simulink model "pidsg"  (R2020a)
settings: Solver=VariableStepAuto  StartTime=0.0  StopTime=0.15  RelTol=1e-3
values from neighbouring files (symbols this model uses):
  aiw_G = 1    [pid_sysgen_v1_0_setup.m]
  f_filter = 5000    [pid_sysgen_v1_0_setup.m]
  FPGA_CLK_MHZ = 125    [pid_sysgen_v1_0_setup.m]
  G1D = (2*R-1)/(2*R+1)    (= 0.995012468828)    [pid_sysgen_v1_0_setup.m]
  G2D = Gd/(2*R+1)    (= 498.753117207)    [pid_sysgen_v1_0_setup.m]
  Gi = ki*Ts/2    (= 1e-06)    [pid_sysgen_v1_0_setup.m]
  input_threshold = 0.0    (= 0)    [pid_sysgen_v1_0_setup.m]
  kd = 0.1    [pid_sysgen_v1_0_setup.m]
  ki = 2    [pid_sysgen_v1_0_setup.m]
  kp = 7    [pid_sysgen_v1_0_setup.m]
  max_control = 0.9    [pid_sysgen_v1_0_setup.m]
  SampleRate = 1e6    (= 1000000)    [pid_sysgen_v1_0_setup.m]
  Ts = 1/SampleRate    (= 1e-06)    [pid_sysgen_v1_0_setup.m]
  VHDL_latency_cycles = 1    [pid_sysgen_v1_0_setup.m]
libraries: xbsIndex_r4 x70, simulink x2
settings Model: Creator=osboxes  LastModifiedBy=valbas

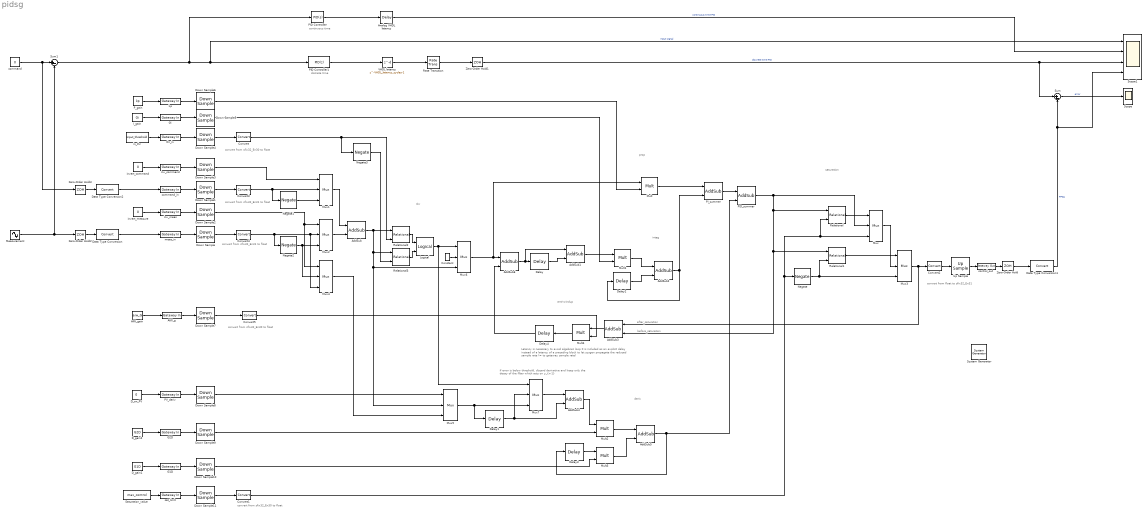
== system pidsg ==
  note: saturation
  note: convert from sfix32_En30 to float
  note: anti-windup
  note: continuous time
  note: before_saturation
  note: integ
  note: thr
  note: prop
  note: if error is below threshold, discard derivative and keep only
      | the decay of the filter which acts on y_{n-1}
  note: Latency is necessary to avoid algebraic loop
      | It is included as an explicit delay instead of a latency of a preceding block
      | to let sysgen propagate the reduced sample rate (= to gateway sample rate)
  note: convert from float to sfix32_En31
  note: convert from sfix32_En30 to float
  note: after_saturation
  note: convert from sfix32_En31 to float
  note: discrete time
  note: convert from sfix32_En31 to float
  note: deriv
  note: convert from sfix32_En30 to float
  " System Generator" : xbsIndex_r4/ System Generator  Tag=genX  xilinxfamily=zynq  part=xc7z030  speed=-1  package=sbg485  synthesis_tool=Vivado  clock_wrapper=Clock Enables  directory=./netlist  proj_type=Vivado  Synth_file=Vivado Synthesis Defaults  Impl_file=Vivado Implementation Defaults  testbench=off  simulink_period=1/(FPGA_CLK_MHZ*1.e6)  sysclk_period=1.e3/FPGA_CLK_MHZ  dcm_input_clock_period=10  incr_netlist=off  trim_vbits=Everywhere in SubSystem  dbl_ovrd=According to Block Masks  core_generation=According to Block Masks  run_coregen=off  deprecated_control=off  eval_field=0  block_type=sysgen
  AIW_g : xbsIndex_r4/Gateway In  gui_display_data_type=Fixed-point  arith_type="Signed  (2's comp)"  n_bits=32  bin_pt=30  preci_type=Single  exp_width=8  frac_width=24  rows=1  columns=1  quantization="Round  (unbiased: +/- Inf)"  overflow=Saturate  period=1/(FPGA_CLK_MHZ*1.e6)  UseAsADC=off  ADCChannel='1'  interface=None  automatic_assignment=on  address_offset=hex2dec('00')  intf_name=''  intf_description=''  default_value=0  timing_constraint=None  locs_specified=off  LOCs={}  io_standard={}  inherit_from_input=off  hdl_port=on  dbl_ovrd=off  block_type=gatewayin
  AIW_gain : Constant  Value=aiw_G  OutDataTypeStr=fixdt(1,32,30)  SampleTime=1/(FPGA_CLK_MHZ*1.e6)
  AddSub : xbsIndex_r4/AddSub  mode=Subtraction  use_carryin=off  use_carryout=off  en=off  latency=0  precision=Full  arith_type=Unsigned  n_bits=16  bin_pt=14  quantization=Truncate  overflow=Wrap  use_behavioral_HDL=off  hw_selection=Fabric  pipelined=off  dbl_ovrd=off  block_type=addsub
  AddSub{1..2,5..6} (4 alike) : xbsIndex_r4/AddSub  mode=Addition  use_carryin=off  use_carryout=off  en=off  latency=0  precision=Full  arith_type=Unsigned  n_bits=16  bin_pt=14  quantization=Truncate  overflow=Wrap  use_behavioral_HDL=off  hw_selection=Fabric  pipelined=off  dbl_ovrd=off  block_type=addsub
  AddSub3 : xbsIndex_r4/AddSub  mode=Subtraction  use_carryin=off  use_carryout=off  en=off  latency=0  precision=Full  arith_type=Unsigned  n_bits=16  bin_pt=14  quantization=Truncate  overflow=Wrap  use_behavioral_HDL=off  hw_selection=Fabric  pipelined=off  dbl_ovrd=off  block_type=addsub
  AddSub4 : xbsIndex_r4/AddSub  mode=Subtraction  use_carryin=off  use_carryout=off  en=off  latency=0  precision=Full  arith_type=Unsigned  n_bits=16  bin_pt=14  quantization=Truncate  overflow=Wrap  use_behavioral_HDL=off  hw_selection=Fabric  pipelined=off  dbl_ovrd=off  block_type=addsub
  Analog VHDL latency : TransportDelay  DelayTime=VHDL_latency_cycles*Ts
  Constant : xbsIndex_r4/Constant  const=0  gui_display_data_type=Floating-point  arith_type=Floating-point  n_bits=16  bin_pt=14  preci_type=Single  exp_width=8  frac_width=24  explicit_period=off  period=1  equ=P=C  opselect=C  inp2=PCIN>>17  opr=+  inp1=P  carry=CIN  dbl_ovrd=off  block_type=constant
  Convert{,1,3..5} (5 alike) : xbsIndex_r4/Convert  gui_display_data_type=Floating-point  arith_type=Floating-point  n_bits=16  bin_pt=14  float_type=Single  exp_bits=8  fraction_bits=24  quantization=Truncate  overflow=Wrap  en=off  latency=0  pipeline=off  dbl_ovrd=off  block_type=convert
  Convert2 : xbsIndex_r4/Convert  gui_display_data_type=Fixed-point  arith_type="Signed  (2's comp)"  n_bits=32  bin_pt=31  float_type=Single  exp_bits=8  fraction_bits=24  quantization="Round  (unbiased: +/- Inf)"  overflow=Saturate  en=off  latency=0  pipeline=off  dbl_ovrd=off  block_type=convert
  D_gain1 : Constant  Value=G1D  OutDataTypeStr=double  SampleTime=1/(FPGA_CLK_MHZ*1.e6)
  D_gain2 : Constant  Value=G2D  OutDataTypeStr=double  SampleTime=1/(FPGA_CLK_MHZ*1.e6)
  D_on_PV : Constant  Value=0  OutDataTypeStr=boolean  SampleTime=1/(FPGA_CLK_MHZ*1.e6)
  Data Type Conversion : DataTypeConversion
  Data Type Conversion1 : DataTypeConversion
  Data Type Conversion2 : DataTypeConversion
  Delay{,1..4} (5 alike) : xbsIndex_r4/Delay  rst=off  infoeditControl=Selection of Reset will increase slice count due to use of real FFs and instead of SRLs  en=off  latency=1  reg_retiming=off  dbl_ovrd=off  block_type=delay
  Down Sample{,1..11} (12 alike) : xbsIndex_r4/Down Sample  sample_ratio=FPGA_CLK_MHZ*1.e6/SampleRate  sample_phase="Last Value of Frame  (most efficient)"  en=off  rst=off  latency=1  dbl_ovrd=off  block_type=dsamp
  G1D : xbsIndex_r4/Gateway In  gui_display_data_type=Floating-point  arith_type=Floating-point  n_bits=16  bin_pt=14  preci_type=Single  exp_width=8  frac_width=24  rows=1  columns=1  quantization="Round  (unbiased: +/- Inf)"  overflow=Saturate  period=1/(FPGA_CLK_MHZ*1.e6)  UseAsADC=off  ADCChannel='1'  interface=None  automatic_assignment=on  address_offset=hex2dec('00')  intf_name=''  intf_description=''  default_value=0  timing_constraint=None  locs_specified=off  LOCs={}  io_standard={}  inherit_from_input=off  hdl_port=on  dbl_ovrd=off  block_type=gatewayin
  G2D : xbsIndex_r4/Gateway In  gui_display_data_type=Floating-point  arith_type=Floating-point  n_bits=16  bin_pt=14  preci_type=Single  exp_width=8  frac_width=24  rows=1  columns=1  quantization="Round  (unbiased: +/- Inf)"  overflow=Saturate  period=1/(FPGA_CLK_MHZ*1.e6)  UseAsADC=off  ADCChannel='1'  interface=None  automatic_assignment=on  address_offset=hex2dec('00')  intf_name=''  intf_description=''  default_value=0  timing_constraint=None  locs_specified=off  LOCs={}  io_standard={}  inherit_from_input=off  hdl_port=on  dbl_ovrd=off  block_type=gatewayin
  Gi : xbsIndex_r4/Gateway In  gui_display_data_type=Floating-point  arith_type=Floating-point  n_bits=16  bin_pt=14  preci_type=Single  exp_width=8  frac_width=24  rows=1  columns=1  quantization="Round  (unbiased: +/- Inf)"  overflow=Saturate  period=1/(FPGA_CLK_MHZ*1.e6)  UseAsADC=off  ADCChannel='1'  interface=None  automatic_assignment=on  address_offset=hex2dec('00')  intf_name=''  intf_description=''  default_value=0  timing_constraint=None  locs_specified=off  LOCs={}  io_standard={}  inherit_from_input=off  hdl_port=on  dbl_ovrd=off  block_type=gatewayin
  I_gain : Constant  Value=Gi  OutDataTypeStr=double  SampleTime=1/(FPGA_CLK_MHZ*1.e6)
  Logical : xbsIndex_r4/Logical  logical_function=OR  inputs=2  en=off  latency=0  precision=Full  arith_type=Unsigned  n_bits=16  bin_pt=0  align_bp=on  dbl_ovrd=off  block_type=logical
  Measurement : Sin  Amplitude=0.1  Frequency=2*pi*17  Phase=0*pi  SampleTime=0
  Mult{,1..4} (5 alike) : xbsIndex_r4/Mult  precision=Full  arith_type="Signed  (2's comp)"  n_bits=16  bin_pt=14  quantization=Truncate  overflow=Wrap  en=off  latency=0  use_behavioral_HDL=off  opt=Speed  use_embedded=on  optimum_pipeline=off  pipeline=on  dbl_ovrd=off  use_rpm=on  placement_style=Triangular  block_type=mult
  Mux{,1..7} (8 alike) : xbsIndex_r4/Mux  inputs=2  en=off  latency=0  precision=Full  arith_type=Unsigned  n_bits=16  bin_pt=14  quantization=Truncate  overflow=Wrap  dbl_ovrd=off  block_type=mux
  Negate{,1..3} (4 alike) : xbsIndex_r4/Negate  precision=Full  arith_type=Unsigned  n_bits=16  bin_pt=14  quantization=Truncate  overflow=Wrap  en=off  latency=0  dbl_ovrd=off  block_type=negate
  PID Controller : simulink/Continuous/PID Controller  Controller=PID  Form=Parallel  TimeDomain=Continuous-time  UseExternalTs=off  SampleTime=-1  IntegratorMethod=Forward Euler  FilterMethod=Forward Euler  ControllerParametersSource=internal  P=kp  I=ki  D=kd  UseFilter=on  N=f_filter  TunerSelectOption=Transfer Function Based (PID Tuner App)  InitialConditionSource=internal  InitialConditionForIntegrator=0  InitialConditionForFilter=0  DifferentiatorICPrevScaledInput=0  ExternalReset=none  TrackingMode=off  Kt=1  LimitOutput=off  UpperSaturationLimit=inf  LowerSaturationLimit=-inf  LinearizeAsGain=on  AntiWindupMode=none  Kb=1  POutMin=[]  POutMax=[]  IOutMin=[]  IOutMax=[]  DOutMin=[]  DOutMax=[]  NOutMin=[]  NOutMax=[]  SumOutMin=[]  SumOutMax=[]  SaturationOutMin=[]  SaturationOutMax=[]  PParamMin=[]  PParamMax=[]  IParamMin=[]  IParamMax=[]  DParamMin=[]  DParamMax=[]  NParamMin=[]  NParamMax=[]  KbParamMin=[]  KbParamMax=[]  KtParamMin=[]  KtParamMax=[]  KbOutMin=[]  KbOutMax=[]  KtOutMin=[]  KtOutMax=[]  IntegratorOutMin=[]  IntegratorOutMax=[]  FilterOutMin=[]  FilterOutMax=[]  SumI1OutMin=[]  SumI1OutMax=[]  SumI2OutMin=[]  SumI2OutMax=[]  SumI3OutMin=[]  SumI3OutMax=[]  SumI4OutMin=[]  SumI4OutMax=[]  SumDOutMin=[]  SumDOutMax=[]  DifferentiatorOutMin=[]  DifferentiatorOutMax=[]  FilterDiffOutCoefMin=[]  FilterDiffOutCoefMax=[]  ReciprocalOutMin=[]  ReciprocalOutMax=[]  SumDenOutMin=[]  SumDenOutMax=[]  SumNumOutMin=[]  SumNumOutMax=[]  DivideOutMin=[]  DivideOutMax=[]  UdiffTsProdOutMin=[]  UdiffTsProdOutMax=[]  NTsProdOutMin=[]  NTsProdOutMax=[]  UintegralTsProdOutMin=[]  UintegralTsProdOutMax=[]  UngainTsProdOutMin=[]  UngainTsProdOutMax=[]  IntegratorContinuousStateAttributes=''  IntegratorStateMustResolveToSignalObject=off  IntegratorRTWStateStorageClass=Auto  FilterContinuousStateAttributes=''  FilterStateMustResolveToSignalObject=off  FilterRTWStateStorageClass=Auto  ParallelPVariant=InternalParameters  IdealPVariant=Disabled  IVariant=InternalParameters  DVariant=InternalParameters  IntegratorVariant=Continuous  SatVariant=Disabled  AWVariant=Passthrough  PCopyVariant=Disabled  TRVariant=Disabled  FdbkBlocksVariant=Forward  IdealPFdbkVariant=Disabled  SatFdbkVariant=Disabled  DerivativeFilterVariant=ContFilter  NVariant=InternalParameters  NCopyVariant=Disabled  FilterICVariant=InternalICsFilter  IntegratorICVariant=InternalICs  ExternalResetVariant=Disabled  TRSumVariant=Passthrough  SumFdbkVariant=Disabled  SumVariant=Sum_PID  TsampFilterVariant=InternalTs  TsampNgainVariant=Passthrough  TsampIntegralVariant=Passthrough
  PID Controller1 : simulink/Continuous/PID Controller  Controller=PID  Form=Parallel  TimeDomain=Discrete-time  UseExternalTs=off  SampleTime=Ts  IntegratorMethod=Trapezoidal  FilterMethod=Trapezoidal  ControllerParametersSource=internal  P=kp  I=ki  D=kd  UseFilter=on  N=f_filter  TunerSelectOption=Transfer Function Based (PID Tuner App)  InitialConditionSource=internal  InitialConditionForIntegrator=0  InitialConditionForFilter=0  DifferentiatorICPrevScaledInput=0  ExternalReset=none  TrackingMode=off  Kt=1  LimitOutput=on  UpperSaturationLimit=max_control  LowerSaturationLimit=-max_control  LinearizeAsGain=on  AntiWindupMode=back-calculation  Kb=aiw_G*ki  POutMin=[]  POutMax=[]  IOutMin=[]  IOutMax=[]  DOutMin=[]  DOutMax=[]  NOutMin=[]  NOutMax=[]  SumOutMin=[]  SumOutMax=[]  SaturationOutMin=[]  SaturationOutMax=[]  PParamMin=[]  PParamMax=[]  IParamMin=[]  IParamMax=[]  DParamMin=[]  DParamMax=[]  NParamMin=[]  NParamMax=[]  KbParamMin=[]  KbParamMax=[]  KtParamMin=[]  KtParamMax=[]  KbOutMin=[]  KbOutMax=[]  KtOutMin=[]  KtOutMax=[]  IntegratorOutMin=[]  IntegratorOutMax=[]  FilterOutMin=[]  FilterOutMax=[]  SumI1OutMin=[]  SumI1OutMax=[]  SumI2OutMin=[]  SumI2OutMax=[]  SumI3OutMin=[]  SumI3OutMax=[]  SumI4OutMin=[]  SumI4OutMax=[]  SumDOutMin=[]  SumDOutMax=[]  DifferentiatorOutMin=[]  DifferentiatorOutMax=[]  FilterDiffOutCoefMin=[]  FilterDiffOutCoefMax=[]  ReciprocalOutMin=[]  ReciprocalOutMax=[]  SumDenOutMin=[]  SumDenOutMax=[]  SumNumOutMin=[]  SumNumOutMax=[]  DivideOutMin=[]  DivideOutMax=[]  UdiffTsProdOutMin=[]  UdiffTsProdOutMax=[]  NTsProdOutMin=[]  NTsProdOutMax=[]  UintegralTsProdOutMin=[]  UintegralTsProdOutMax=[]  UngainTsProdOutMin=[]  UngainTsProdOutMax=[]  IntegratorContinuousStateAttributes=''  IntegratorStateMustResolveToSignalObject=off  IntegratorRTWStateStorageClass=Auto  FilterContinuousStateAttributes=''  FilterStateMustResolveToSignalObject=off  FilterRTWStateStorageClass=Auto  ParallelPVariant=InternalParameters  IdealPVariant=Disabled  IVariant=InternalParameters  DVariant=InternalParameters  IntegratorVariant=Discrete  SatVariant=Enabled  AWVariant=BackCalculation  PCopyVariant=Disabled  TRVariant=Disabled  FdbkBlocksVariant=Feedback  IdealPFdbkVariant=Passthrough  SatFdbkVariant=Enabled  DerivativeFilterVariant=TrapezoidalFilter  NVariant=InternalParameters  NCopyVariant=InternalParameters  FilterICVariant=InternalICsFilter  IntegratorICVariant=InternalICs  ExternalResetVariant=Disabled  TRSumVariant=Passthrough  SumFdbkVariant=Enabled  SumVariant=Sum_PID  TsampFilterVariant=InternalTs  TsampNgainVariant=Passthrough  TsampIntegralVariant=Passthrough
  PID_summer : xbsIndex_r4/AddSub  mode=Addition  use_carryin=off  use_carryout=off  en=off  latency=0  precision=Full  arith_type=Unsigned  n_bits=16  bin_pt=14  quantization=Truncate  overflow=Wrap  use_behavioral_HDL=off  hw_selection=Fabric  pipelined=off  dbl_ovrd=off  block_type=addsub
  PI_summer : xbsIndex_r4/AddSub  mode=Addition  use_carryin=off  use_carryout=off  en=off  latency=0  precision=Full  arith_type=Unsigned  n_bits=16  bin_pt=14  quantization=Truncate  overflow=Wrap  use_behavioral_HDL=off  hw_selection=Fabric  pipelined=off  dbl_ovrd=off  block_type=addsub
  PV_deriv : xbsIndex_r4/Gateway In  gui_display_data_type=Boolean  arith_type=Boolean  n_bits=16  bin_pt=14  preci_type=Single  exp_width=8  frac_width=24  rows=1  columns=1  quantization="Round  (unbiased: +/- Inf)"  overflow=Saturate  period=1/(FPGA_CLK_MHZ*1.e6)  UseAsADC=off  ADCChannel='1'  interface=None  automatic_assignment=on  address_offset=hex2dec('00')  intf_name=''  intf_description=''  default_value=0  timing_constraint=None  locs_specified=off  LOCs={}  io_standard={}  inherit_from_input=off  hdl_port=on  dbl_ovrd=off  block_type=gatewayin
  P_gain : Constant  Value=kp  OutDataTypeStr=double  SampleTime=1/(FPGA_CLK_MHZ*1.e6)
  Rate Transition : RateTransition  OutPortSampleTime=1/(FPGA_CLK_MHZ*1.e6)
  Relational : xbsIndex_r4/Relational  mode=a>b  op_type=Bool  en=off  latency=0  dbl_ovrd=off  block_type=relational
  Relational1 : xbsIndex_r4/Relational  mode=a<b  op_type=Bool  en=off  latency=0  dbl_ovrd=off  block_type=relational
  Relational2 : xbsIndex_r4/Relational  mode=a>b  op_type=Bool  en=off  latency=0  dbl_ovrd=off  block_type=relational
  Relational3 : xbsIndex_r4/Relational  mode=a<b  op_type=Bool  en=off  latency=0  dbl_ovrd=off  block_type=relational
  Saturation_value : Constant  Value=max_control  OutDataTypeStr=fixdt(1,32,30)  SampleTime=1/(FPGA_CLK_MHZ*1.e6)
  Scope : Scope
  Scope1 : Scope  NumInputPorts=4
  Sum : Sum  Inputs=|+-
  Sum1 : Sum  Inputs=|+-
  Up Sample : xbsIndex_r4/Up Sample  sample_ratio=FPGA_CLK_MHZ*1.e6/SampleRate  copy_samples=on  en=off  latency=1  dbl_ovrd=off  block_type=usamp
  VHDL latency : Delay  DelayLength=VHDL_latency_cycles-1
  Zero-Order Hold{,1..3} (4 alike) : ZeroOrderHold  SampleTime=1/(FPGA_CLK_MHZ*1.e6)
  command : Constant  Value=0  OutDataTypeStr=double  SampleTime=0
  command_in : xbsIndex_r4/Gateway In  gui_display_data_type=Fixed-point  arith_type="Signed  (2's comp)"  n_bits=32  bin_pt=31  preci_type=Single  exp_width=8  frac_width=24  rows=1  columns=1  quantization="Round  (unbiased: +/- Inf)"  overflow=Saturate  period=1/(FPGA_CLK_MHZ*1.e6)  UseAsADC=off  ADCChannel='1'  interface=None  automatic_assignment=on  address_offset=hex2dec('00')  intf_name=''  intf_description=''  default_value=0  timing_constraint=None  locs_specified=off  LOCs={}  io_standard={}  inherit_from_input=off  hdl_port=on  dbl_ovrd=off  block_type=gatewayin
  control_out : xbsIndex_r4/Gateway Out  inherit_from_input=on  hdl_port=on  rows=1  columns=1  UseAsDAC=off  DACChannel='1'  interface=None  automatic_assignment=on  address_offset=hex2dec('00')  intf_name=''  intf_description=''  timing_constraint=Data Rate  locs_specified=off  LOCs={}  io_standard={}  block_type=gatewayout
  in_thr : Constant  Value=input_threshold  OutDataTypeStr=fixdt(1,32,30)  SampleTime=1/(FPGA_CLK_MHZ*1.e6)
  inv_command : xbsIndex_r4/Gateway In  gui_display_data_type=Boolean  arith_type=Boolean  n_bits=16  bin_pt=14  preci_type=Single  exp_width=8  frac_width=24  rows=1  columns=1  quantization="Round  (unbiased: +/- Inf)"  overflow=Saturate  period=1/(FPGA_CLK_MHZ*1.e6)  UseAsADC=off  ADCChannel='1'  interface=None  automatic_assignment=on  address_offset=hex2dec('00')  intf_name=''  intf_description=''  default_value=0  timing_constraint=None  locs_specified=off  LOCs={}  io_standard={}  inherit_from_input=off  hdl_port=on  dbl_ovrd=off  block_type=gatewayin
  inv_meas : xbsIndex_r4/Gateway In  gui_display_data_type=Boolean  arith_type=Boolean  n_bits=16  bin_pt=14  preci_type=Single  exp_width=8  frac_width=24  rows=1  columns=1  quantization="Round  (unbiased: +/- Inf)"  overflow=Saturate  period=1/(FPGA_CLK_MHZ*1.e6)  UseAsADC=off  ADCChannel='1'  interface=None  automatic_assignment=on  address_offset=hex2dec('00')  intf_name=''  intf_description=''  default_value=0  timing_constraint=None  locs_specified=off  LOCs={}  io_standard={}  inherit_from_input=off  hdl_port=on  dbl_ovrd=off  block_type=gatewayin
  invert_command : Constant  Value=0  OutDataTypeStr=boolean  SampleTime=1/(FPGA_CLK_MHZ*1.e6)
  invert_measure : Constant  Value=0  OutDataTypeStr=boolean  SampleTime=1/(FPGA_CLK_MHZ*1.e6)
  kp : xbsIndex_r4/Gateway In  gui_display_data_type=Floating-point  arith_type=Floating-point  n_bits=16  bin_pt=14  preci_type=Single  exp_width=8  frac_width=24  rows=1  columns=1  quantization="Round  (unbiased: +/- Inf)"  overflow=Saturate  period=1/(FPGA_CLK_MHZ*1.e6)  UseAsADC=off  ADCChannel='1'  interface=None  automatic_assignment=on  address_offset=hex2dec('00')  intf_name=''  intf_description=''  default_value=0  timing_constraint=None  locs_specified=off  LOCs={}  io_standard={}  inherit_from_input=off  hdl_port=on  dbl_ovrd=off  block_type=gatewayin
  meas_in : xbsIndex_r4/Gateway In  gui_display_data_type=Fixed-point  arith_type="Signed  (2's comp)"  n_bits=32  bin_pt=31  preci_type=Single  exp_width=8  frac_width=24  rows=1  columns=1  quantization="Round  (unbiased: +/- Inf)"  overflow=Saturate  period=1/(FPGA_CLK_MHZ*1.e6)  UseAsADC=off  ADCChannel='1'  interface=None  automatic_assignment=on  address_offset=hex2dec('00')  intf_name=''  intf_description=''  default_value=0  timing_constraint=None  locs_specified=off  LOCs={}  io_standard={}  inherit_from_input=off  hdl_port=on  dbl_ovrd=off  block_type=gatewayin
  sat_limit : xbsIndex_r4/Gateway In  gui_display_data_type=Fixed-point  arith_type="Signed  (2's comp)"  n_bits=32  bin_pt=30  preci_type=Single  exp_width=8  frac_width=24  rows=1  columns=1  quantization="Round  (unbiased: +/- Inf)"  overflow=Saturate  period=1/(FPGA_CLK_MHZ*1.e6)  UseAsADC=off  ADCChannel='1'  interface=None  automatic_assignment=on  address_offset=hex2dec('00')  intf_name=''  intf_description=''  default_value=0  timing_constraint=None  locs_specified=off  LOCs={}  io_standard={}  inherit_from_input=off  hdl_port=on  dbl_ovrd=off  block_type=gatewayin
  thr_in : xbsIndex_r4/Gateway In  gui_display_data_type=Fixed-point  arith_type="Signed  (2's comp)"  n_bits=32  bin_pt=30  preci_type=Single  exp_width=8  frac_width=24  rows=1  columns=1  quantization="Round  (unbiased: +/- Inf)"  overflow=Saturate  period=1/(FPGA_CLK_MHZ*1.e6)  UseAsADC=off  ADCChannel='1'  interface=None  automatic_assignment=on  address_offset=hex2dec('00')  intf_name=''  intf_description=''  default_value=0  timing_constraint=None  locs_specified=off  LOCs={}  io_standard={}  inherit_from_input=off  hdl_port=on  dbl_ovrd=off  block_type=gatewayin
  wires:
  Data Type Conversion1/1 -> Scope1/4, Sum/2  "FPGA"
  Relational2/1 -> Logical/1
  Convert/1 -> Negate3/1, Relational2/2
  Negate/1 -> Mux3/3, Relational1/2
  PID Controller1/1 -> VHDL latency/1
  Data Type Conversion2/1 -> command_in/1
  Mux6/1 -> AddSub6/1, Mult/1
  Mux4/1 -> Mux5/3
  Negate1/1 -> Mux1/3
  Mux/1 -> Mux3/2
  Mult2/1 -> AddSub5/1
  Mux7/1 -> AddSub4/1
  Relational3/1 -> Logical/2
  invert_command/1 -> inv_command/1
  command/1 -> Zero-Order Hold3/1, Sum1/1
  Mux2/1 -> AddSub/2
  Logical/1 -> Mux7/1, Mux6/1
  Data Type Conversion/1 -> meas_in/1
  thr_in/1 -> Down Sample4/1
  AddSub2/1 -> Delay2/1, PI_summer/2
  meas_in/1 -> Down Sample/1
  Negate3/1 -> Relational3/2
  Convert1/1 -> Relational/2, Mux/3, Negate/1
  Delay2/1 -> AddSub2/2
  AddSub1/1 -> Mult1/1
  Constant/1 -> Mux6/2
  Negate2/1 -> Mux4/2, Mux2/3
  Delay1/1 -> Mux7/2, AddSub4/2
  D_gain1/1 -> G1D/1
  Mux3/1 -> Convert2/1, AddSub3/1
  control_out/1 -> Zero-Order Hold/1
  Mux5/1 -> Mux7/3, Delay1/1
  AddSub3/1 -> Mult4/1
  Relational1/1 -> Mux3/1
  PID Controller/1 -> Analog VHDL latency/1
  Delay3/1 -> Mult3/1
  Convert3/1 -> Negate1/1, Mux1/2
  Mult/1 -> PI_summer/1
  AddSub4/1 -> Mult2/1
  inv_command/1 -> Down Sample3/1
  in_thr/1 -> thr_in/1
  AddSub5/1 -> PID_summer/2, Delay3/1
  Delay4/1 -> AddSub6/2
  Mux1/1 -> AddSub/1
  kp/1 -> Down Sample6/1
  G1D/1 -> Down Sample10/1
  AIW_g/1 -> Down Sample7/1
  sat_limit/1 -> Down Sample11/1
  AddSub/1 -> Relational2/1, Relational3/1, Mux6/3, Mux5/2
  Convert4/1 -> Mux4/3, Mux2/2, Negate2/1
  Relational/1 -> Mux/1
  Mult3/1 -> AddSub5/2
  D_on_PV/1 -> PV_deriv/1
  G2D/1 -> Down Sample9/1
  Delay/1 -> AddSub1/2
  Mult1/1 -> AddSub2/1
  PV_deriv/1 -> Down Sample8/1
  Analog VHDL latency/1 -> Scope1/2  "continuous time PID"
  PID_summer/1 -> Mux/2, AddSub3/2, Relational1/1, Relational/1
  AIW_gain/1 -> AIW_g/1
  invert_measure/1 -> inv_meas/1
  Mult4/1 -> Delay4/1
  P_gain/1 -> kp/1
  PI_summer/1 -> PID_summer/1
  I_gain/1 -> Gi/1
  Gi/1 -> Down Sample5/1
  Sum/1 -> Scope/1  "error"
  Sum1/1 -> Scope1/1, PID Controller1/1, PID Controller/1  "input signal"
  Saturation_value/1 -> sat_limit/1
  VHDL latency/1 -> Rate Transition/1
  Measurement/1 -> Zero-Order Hold2/1, Sum1/2
  command_in/1 -> Down Sample1/1
  D_gain2/1 -> G2D/1
  inv_meas/1 -> Down Sample2/1
  AddSub6/1 -> AddSub1/1, Delay/1
  Convert5/1 -> Mult4/2
  Convert2/1 -> Up Sample/1
  Up Sample/1 -> control_out/1
  Zero-Order Hold/1 -> Data Type Conversion1/1
  Zero-Order Hold1/1 -> Sum/1, Scope1/3  "discrete time PID"
  Zero-Order Hold2/1 -> Data Type Conversion/1
  Zero-Order Hold3/1 -> Data Type Conversion2/1
  Rate Transition/1 -> Zero-Order Hold1/1
  Down Sample/1 -> Convert4/1
  Down Sample1/1 -> Convert3/1
  Down Sample2/1 -> Mux4/1, Mux2/1
  Down Sample3/1 -> Mux1/1
  Down Sample4/1 -> Convert/1
  Down Sample5/1 -> Mult1/2
  Down Sample6/1 -> Mult/2
  Down Sample7/1 -> Convert5/1
  Down Sample8/1 -> Mux5/1
  Down Sample9/1 -> Mult2/2
  Down Sample10/1 -> Mult3/2
  Down Sample11/1 -> Convert1/1
